simulink subsystem "Magnetometer_MMC5983MA"  (R2025b)
settings: Solver=VariableStepAuto  StartTime=0.0  StopTime=10.0  RelTol=1e-3
undefined symbols (not defined in the file): mag_sensor
settings Model: Creator=slee7  LastModifiedBy=Admin

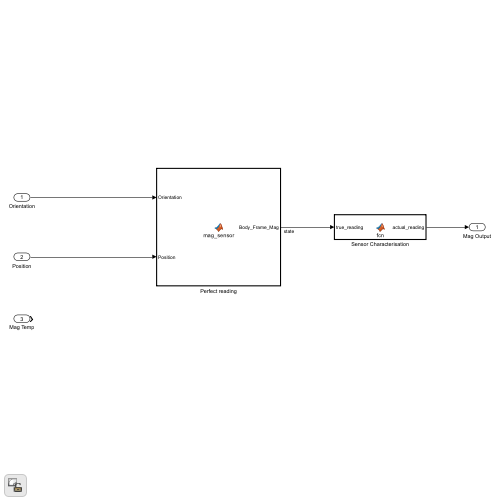
[thumbnail: Simulink's stored preview of the top-level diagram]
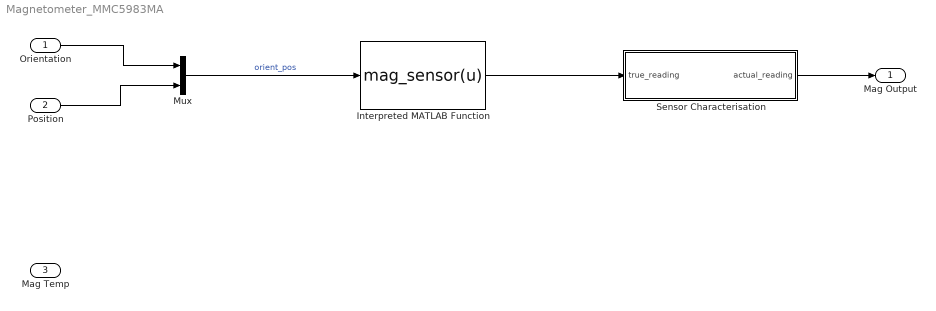
== system Magnetometer_MMC5983MA ==
  Orientation : Inport
  Position : Inport  Port=2
  Mag Temp : Inport  Port=3
  Interpreted MATLAB Function : MATLABFcn  MATLABFcn=mag_sensor(u)  OutputDimensions=[6 1]  OutputSignalType=real  Output1D=off
  Mux : Mux  Inputs=2
  Sensor Characterisation : MATLAB Function  TreatAsAtomicUnit=on
  Mag Output : Outport
  wires:
  Sensor Characterisation/1(actual_reading) -> Mag Output/1
  Orientation/1 -> Mux/1
  Position/1 -> Mux/2
  Mux/1 -> Interpreted MATLAB Function/1  "orient_pos"
  Interpreted MATLAB Function/1 -> Sensor Characterisation/1(true_reading)

== matlab function Magnetometer_MMC5983MA/Sensor Characterisation ==
  data: true_reading input; actual_reading output
function actual_reading = fcn(true_reading)
    persistent b_previous

    % Spherical Calibration
   
    b = [-0.0705; -0.1152; 0.0250];
    A = [2.2439, -0.0154, -0.0144;
        -0.0154, 2.2042, -0.097;
        -0.0144, -0.0097, 2.4001];

    % Hard-Iron Bias (Offset)
    cal_reading = true_reading(1:3) - b;

    % Soft-Iron Bias (Scale Distortion)
    cal_reading = A * cal_reading;


    dt = 0.02; % CAN Bus limit 20 ms
    % Simulation Time Step for BW=11 (Measurement Time): 0.0005

    % Bias: Composite Bias = Const + Gauss-Markov Drift
    
        b_const = [0; 0; 0]; % Constant bias
    
        % Drift bias b_{k+1} &= e^{-\Delta t/ \tau} * b_k + \omega_k
        
        if isempty(b_previous)
            b_previous = [0; 0; 0]; 
        end
    
        tau = [6.9630; 7.8914; 6.3777]; % time constant of drift
        q = [1.1384e-11; 2.9369e-11; 4.0735e-11]; % variance on drift
    
        omega = sqrt(q) .* randn(3,1); % omega ~ N(0,q)
        
        phi = exp(-dt ./ tau);
        b_drift = phi .* b_previous + omega;

        b_previous = b_drift;
    
        composite_bias = b_const + b_drift; 

    % Noise: Gaussian

        noise_std = [1.2; 1.2; 1.2];      % [Total RMS Noise for BW=11]
    
        noise = noise_std .* randn(3,1); % noise ~ N(0,noise_variance)
    
    % Quantisation:

        quant_step = [0.0625; 0.0625; 0.0625]; % Quant Step (for 18-bit)
   

    % Reading Processing:

        actual_reading_continuous  = cal_reading(:) + composite_bias + noise;

        actual_reading_quantised = quant_step .* round(actual_reading_continuous./quant_step);

        actual_reading = [actual_reading_quantised; true_reading(4:6)];

end

% Currently Ignoring: 
% Scale_factor_error 
% Misalignment_error
